simulink model "dcdrive"  (Simulink 5.0)
settings: Solver=ode15s  SolverMode=SingleTasking  StartTime=0.0  StopTime=2.5
libraries: powerlib2 x12
settings Model: ExtModeTrigMode=oneshot  ExtModeArmWhenConnect=off  SaveTime=off  SaveOutput=off  SaveFinalState=on  LimitDataPoints=off  UnconnectedInputMsg=none  UnconnectedOutputMsg=none  BlockReductionOpt=off  BooleanDataType=off  RTWTemplateMakefile=grt_unix.tmf

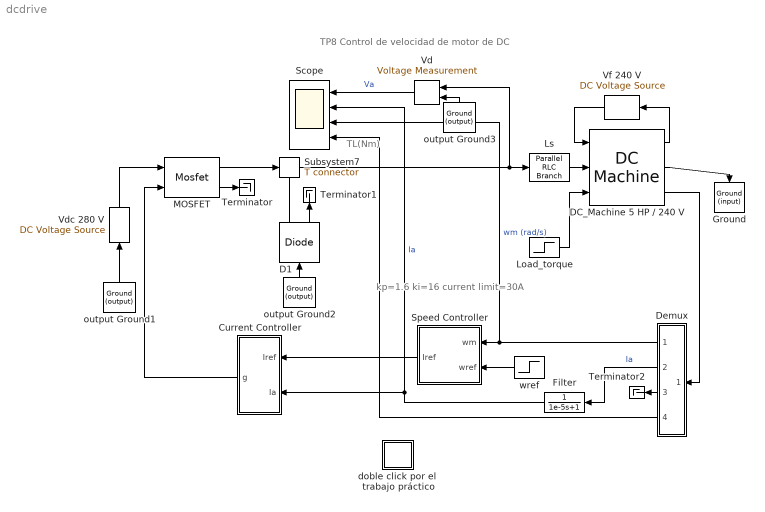
== system dcdrive ==
  note: TL(Nm)
  note: TP8 Control de velocidad de motor de DC
  note: kp=1.6
      | ki=16
      | current limit=30A
  Current Controller : Subsystem  Orientation=left  mask{h=2}
      mask prompts: h "Hysteresis band (A)"
      mask help: Hysteresis Current Controller
      mask Display: plot(0,0,100,100,[45,45],[35,65],[55,55],[35,65],[45,65],[65,65],[35,55],[35,35])
  D1 : powerlib2/Power Electronics/Diode  Tag=PoWeRsYsTeMbLoCk  Orientation=up  Ron=0.05  Lon=5e-6  Vf=0.7  IC=0  Rs=Inf  Cs=0.1e-6  PSBOutputType=10
  DC_Machine 5 HP / 240 V : powerlib2/Machines/DC Machine  RLa="[0.5  0.01]"  RLf="[240  0]"  Laf=1.23  J=0.05  Bm=0.02  Tf=0  w0=1e-1  PSBOutputType=110
  Demux : Subsystem  Orientation=left
  Filter : TransferFcn  Orientation=left  Numerator=1  Denominator=[1e-5 1]
      mask Display: disp('Filter')
  Ground : powerlib2/Connectors/Ground (input)  Tag=PoWeRsYsTeMbLoCk  Orientation=down
  "Load_torque " : Step  Time=1.2  Before=5  After=25  SampleTime=0
  Ls : powerlib2/Elements/Parallel RLC Branch  Tag=PoWeRsYsTeMbLoCk  a=inf  b=10e-03  c=0  mesure=None  PSBOutputType=1
  MOSFET : powerlib2/Power Electronics/Mosfet  Tag=PoWeRsYsTeMbLoCk  Ron=0.001  Lon=1e-6  Rd=.001  IC=0  Rs=10  Cs=0.01e-6  PSBOutputType=10
  Scope : Scope  NumInputPorts=4
      settings: TickLabels=on  YMin=-600~0~100~0  YMax=400~35~180~40  SaveName=var  Decimation=20
  Speed Controller : Subsystem  Orientation=left  mask(PI controller){Kp=1.6, Ki=16, Ilim=30}
      mask prompts: Kp "Proportional gain (Kp)"; Ki "Integral gain (Ki)"; Ilim "Current limit (A)"
      mask help: Proportional-Integral Speed Controller
      mask Display: plot(0,0,100,100,[35,35,65],[70,30,30],[35,65],[45,60])
  Subsystem7 : powerlib2/Connectors/T connector  Tag=PoWeRsYsTeMbLoCk  PSBOutputType=1
  Terminator : Terminator
  Terminator1 : Terminator
      settings: Orientation=up
  Terminator2 : Terminator
  Vd : powerlib2/Measurements/Voltage Measurement  Tag=PoWeRsYsTeMmEaSuReMeNt  Orientation=left  PhasorSimulation=off  OutputType=Magnitude  PSBOutputType=0  PSBequivalent=1
  "Vdc 280 V " : powerlib2/Electrical Sources/DC Voltage Source  Tag=PoWeRsYsTeMbLoCk  Orientation=up  V=280  mesure=None  PSBOutputType=1
  Vf 240 V : powerlib2/Electrical Sources/DC Voltage Source  Tag=PoWeRsYsTeMbLoCk  Orientation=left  V=240  mesure=None  PSBOutputType=1
  doble click por el  trabajo práctico : Subsystem
      mask Display: disp('?')
  output Ground1 : powerlib2/Connectors/Ground (output)  Tag=PoWeRsYsTeMbLoCk  Orientation=up  PSBOutputType=1
  output Ground2 : powerlib2/Connectors/Ground (output)  Tag=PoWeRsYsTeMbLoCk  Orientation=up  PSBOutputType=1
  output Ground3 : powerlib2/Connectors/Ground (output)  Tag=PoWeRsYsTeMbLoCk  Orientation=up  PSBOutputType=1
  "wref " : Step  Orientation=left  Time=0.4  Before=120  After=160  SampleTime=0
  wires:
  D1/2 -> Terminator1/1
  MOSFET/2 -> Terminator/1
  output Ground2/1 -> D1/1
  D1/1 -> Subsystem7/Enable
  MOSFET/1 -> Subsystem7/1
  Current Controller/1(g) -> MOSFET/2
  "Vdc 280 V "/1 -> MOSFET/1
  output Ground1/1 -> "Vdc 280 V "/1
  Ls/1 -> DC_Machine 5 HP / 240 V/2
  Vf 240 V/1 -> DC_Machine 5 HP / 240 V/1
  Vd/1 -> Scope/1  "Va"
  Speed Controller/1(Iref) -> Current Controller/1(Iref)
  Subsystem7/1 -> Ls/1, Vd/1
  output Ground3/1 -> Vd/2
  Filter/1 -> Current Controller/2(Ia), Scope/2  "Ia"
  DC_Machine 5 HP / 240 V/2 -> Ground/1
  DC_Machine 5 HP / 240 V/1 -> Vf 240 V/1
  DC_Machine 5 HP / 240 V/3 -> Demux/1(m)
  Demux/2(Ia) -> Filter/1  "Ia"
  Demux/4(Te) -> Scope/4
  Demux/3(If) -> Terminator2/1
  "Load_torque "/1 -> DC_Machine 5 HP / 240 V/3
  "wref "/1 -> Speed Controller/2(wref)
  Demux/1(wm) -> Speed Controller/1(wm), Scope/3  "wm (rad/s)"

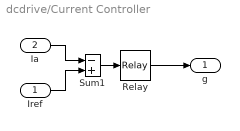
== system dcdrive/Current Controller ==
  Iref : Inport
  Ia : Inport  Port=2
  Relay : Relay  OnSwitchValue=h/2  OffSwitchValue=-h/2  OnOutputValue=10
  Sum1 : Sum  Inputs=-+  SaturateOnIntegerOverflow=on  InputSameDT=on
  g : Outport  InitialOutput=0
  wires:
  Sum1/1 -> Relay/1
  Relay/1 -> g/1
  Ia/1 -> Sum1/1
  Iref/1 -> Sum1/2

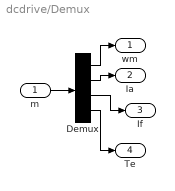
== system dcdrive/Demux ==
  m : Inport
  Demux : Demux
  wm : Outport
  Ia : Outport  Port=2
  If : Outport  Port=3
  Te : Outport  Port=4
  wires:
  Demux/1 -> wm/1
  Demux/2 -> Ia/1
  m/1 -> Demux/1
  Demux/3 -> If/1
  Demux/4 -> Te/1

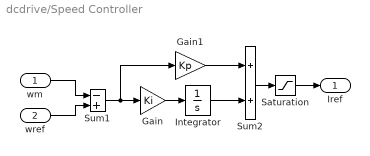
== system dcdrive/Speed Controller ==
  wm : Inport
  wref : Inport  Port=2
  Gain : Gain  Gain=Ki  SaturateOnIntegerOverflow=on
  Gain1 : Gain  Gain=Kp  SaturateOnIntegerOverflow=on
  Integrator : Integrator  LimitOutput=on  UpperSaturationLimit=Ilim  LowerSaturationLimit=-Ilim
  Saturation : Saturate  UpperLimit=Ilim  LowerLimit=-Ilim
  Sum1 : Sum  Inputs=-+  SaturateOnIntegerOverflow=on  InputSameDT=on
  Sum2 : Sum  SaturateOnIntegerOverflow=on  InputSameDT=on
  Iref : Outport  InitialOutput=0
  wires:
  Saturation/1 -> Iref/1
  Sum2/1 -> Saturation/1
  Integrator/1 -> Sum2/2
  wref/1 -> Sum1/2
  wm/1 -> Sum1/1
  Sum1/1 -> Gain1/1, Gain/1
  Gain/1 -> Integrator/1
  Gain1/1 -> Sum2/1

== system dcdrive/doble click por el  trabajo práctico ==
  note: Ejecute la simulación. Observe en el osciloscopio la tensión del motor, corriente, velocidad y par.
      |
      | La referencia de velocidad es un escalón que comienza con wm = 120 rad/s y en el instante de tiempo (0,4s)
      | cambia por wm = 120 rad/s.
      |
      | El par cambia con forma de escalón desde el valor inicial TL = 5 N.m a Te = 25 N.m en 1,2 seg.
  note: TP 8; Case study I: Chopper-Fed DC Motor Drive
  note: Circuit description
  note: Womework
  note: El motor de DC está alimentado por un chopper de DC con MOSFET operando en clase A.
      | La carga mecánica está caracterizada por un escalón de carga TL.
      |
      | El controlador de corriente de histéresis compara la corriente sensada con una referencia y genera la señal de compuerta
      | del MOSFET forzando al motor a seguir la corriente de referencia.
      | El lazo de velocidad utiliza un controlador PI que produce la referencia para el lazo de corriente (par).
      | El bloque de Voltage Measurement provee señal para los propositos de visualización.
  note: (Modificado del archivo original de H. Le-Huy, Université Laval, Québec)
  note: Measurements
  note: a) Imprima las magnitudes medidas en osciloscopio
      | b) Mida la constante de tiempo eléctrica del motor
      | c) Mida la constante de tiempo mecánica del motor
      | d) Cambie los valores del controlador (speed controller)
      | y busque (prueba y error) la sintonización más óptima,
      | sin cambiar el límite de corriente.
  note: Conclusion
  note: a) acerca de las constantes de tiempo
      | b) acerca de la ecuación general de par Te=TL+J*d(wm)/dt
      | c) Acerca del controlador (speed controller)
      | d) generales (otros)
